simulink model "case_07_slow_sine_wave_then_accelerate"  (R2025b)
settings: Solver=VariableStepAuto  StartTime=0.0  StopTime=120  RelTol=1e-3
settings Model: Creator=sanborkl  LastModifiedBy=sanborkl

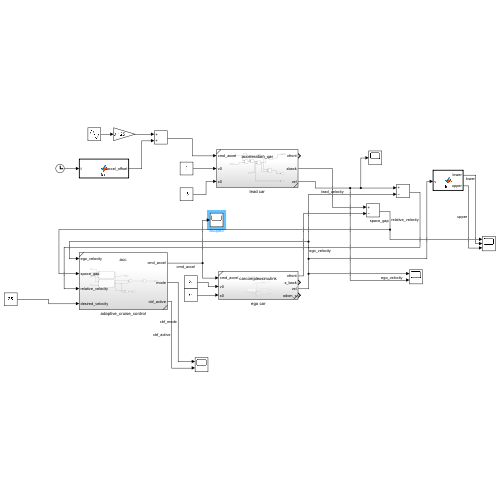
[thumbnail: Simulink's stored preview of the top-level diagram]
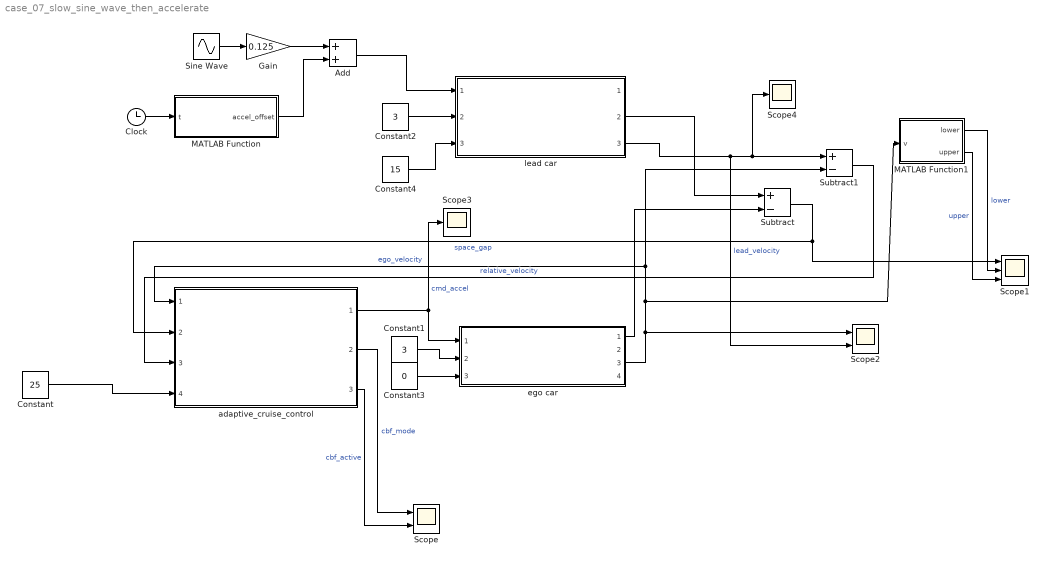
== system case_07_slow_sine_wave_then_accelerate ==
  Add : Sum
  Clock : Clock
  Constant : Constant  Value=25
  Constant1 : Constant  Value=3
  Constant2 : Constant  Value=3
  Constant3 : Constant  Value=0
  Constant4 : Constant  Value=15
  Gain : Gain  Gain=0.125
  MATLAB Function : MATLAB Function  TreatAsAtomicUnit=on
  MATLAB Function1 : MATLAB Function  TreatAsAtomicUnit=on
  Scope : Scope  NumInputPorts=2
      settings: ActiveDisplayYMinimum=0.75000000000000011  ActiveDisplayYMaximum=3.25
  Scope1 : Scope  NumInputPorts=3
      settings: ActiveDisplayYMinimum=-7.5554081669496682  ActiveDisplayYMaximum=160.0434581700147  YLabel=m
  Scope2 : Scope  NumInputPorts=2
      settings: ActiveDisplayYMinimum=-1.9876142444183507  ActiveDisplayYMaximum=38.910920533498995  YLabel=m/s  DataLoggingVariableName=ScopeData2
  Scope3 : Scope
      settings: ActiveDisplayYMinimum=-1.310508335295592  ActiveDisplayYMaximum=1.1945750176603234  YLabel=m/s^2  DataLoggingVariableName=ScopeData3
  Scope4 : Scope
      settings: ActiveDisplayYMinimum=-1  ActiveDisplayYMaximum=1  DataLoggingVariableName=ScopeData4
  Sine Wave : Sin  Frequency=0.125  SampleTime=0
  Subtract : Sum  Inputs=+-
  Subtract1 : Sum  Inputs=+-
  adaptive_cruise_control : Subsystem  ReferencedSubsystem=acc
  ego car : Subsystem  ReferencedSubsystem=carcomplexsimulink
  lead car : Subsystem  ReferencedSubsystem=acceleration_car
  wires:
  ego car/3 -> Subtract1/2, adaptive_cruise_control/1, MATLAB Function1/1(v), Scope2/1  "ego_velocity"
  adaptive_cruise_control/1 -> ego car/1, Scope3/1  "cmd_accel"
  Constant1/1 -> ego car/2
  Subtract1/1 -> adaptive_cruise_control/3  "relative_velocity"
  lead car/3 -> Scope2/2, Scope4/1, Subtract1/1  "lead_velocity"
  Constant3/1 -> ego car/3
  Constant2/1 -> lead car/2
  adaptive_cruise_control/2 -> Scope/1  "cbf_mode"
  lead car/2 -> Subtract/1
  adaptive_cruise_control/3 -> Scope/2  "cbf_active"
  Constant/1 -> adaptive_cruise_control/4
  ego car/1 -> Subtract/2
  Subtract/1 -> Scope1/1, adaptive_cruise_control/2  "space_gap"
  Constant4/1 -> lead car/3
  Sine Wave/1 -> Gain/1
  MATLAB Function/1(accel_offset) -> Add/2
  Add/1 -> lead car/1
  Clock/1 -> MATLAB Function/1(t)
  Gain/1 -> Add/1
  MATLAB Function1/1(lower) -> Scope1/2  "lower"
  MATLAB Function1/2(upper) -> Scope1/3  "upper"

== matlab function case_07_slow_sine_wave_then_accelerate/MATLAB Function ==
  data: t input; accel_offset output
function accel_offset = fcn(t)

if t <= 60
    accel_offset = 0;
else
    accel_offset = 0.5;
end

== matlab function case_07_slow_sine_wave_then_accelerate/MATLAB Function1 ==
  data: v input; lower output; upper output
function [lower, upper] = fcn(v)

lower = 2 * v + 5;
upper = 2 * v + 15;
